simulink model "VisualLocalizationAgent"  (R2024b)
settings: Solver=VariableStepAuto  StartTime=0.0  StopTime=inf  FixedStep=0.05  RelTol=1e-3  EnableMultiTasking=on
undefined symbols (not defined in the file or in its folder): gray, Sim3dSensor
libraries: robotcorelib x2, sim3dcameralib x1, sim3dlib x1, uavsim3dlib x1, uavutilslib x1
settings Model: Creator=The MathWorks, Inc.  LastModifiedBy=vince
settings SolverCC: AlgebraicLoopSolver=TrustRegion  PositivePriorityOrder=on  AutoInsertRateTranBlk=on  MaxZcPerStep=1
settings OptimizationCC: DefaultParameterBehavior=Inlined  EnhancedBackFolding=on  PassReuseOutputArgsAs=Individual arguments  ZeroExternalMemoryAtStartup=off  ZeroInternalMemoryAtStartup=off  MaxStackSize=200000  OptimizeBlockOrder=speed  DifferentSizesBufferReuse=on  OptimizationCustomize=off  EfficientTunableParamExpr=on
settings DebuggingCC: ParameterTunabilityLossMsg=error  UnconnectedInputMsg=warning  UnconnectedOutputMsg=warning  UnconnectedLineMsg=warning  SymbolicDimsDataTypeCodeGenerationDiagnostic=none
settings HardwareCC: ProdBitPerPointer=32  ProdBitPerSizeT=32  ProdBitPerPtrDiffT=32  ProdLargestAtomicInteger=Long  ProdLargestAtomicFloat=Double  ProdWordSize=32  ProdLongLongMode=on  ProdHWDeviceType=ARM Compatible->ARM Cortex-A (32-bit)
settings ModelReferenceCC: EnableRefExpFcnMdlSchedulingChecks=on
settings RTWCC: Description=Embedded Coder  SystemTargetFile=ert.tlc  HardwareBoard=Raspberry Pi  TLCOptions="-aInlineSetEventsForThisBaseRateFcn=TLC_FALSE -aSuppressMultiTaskScheduler=TLC_FALSE  -aRateBasedStepFcn=0"  TemplateMakefile=ert_default_tmf  Toolchain=GNU GCC Embedded Linux  BuildConfiguration=Faster Runs  GPUComputeCapability=3.5  DLArmComputeVersion=19.05
settings CodeAppCC: ForceParamTrailComments=on  IgnoreCustomStorageClasses=off  OperatorAnnotations=on  SimulinkDataObjDesc=on  SFDataObjDesc=on  InsertBlockDesc=on
settings ERTTargetCC: CodeReplacementLibrary=ARM Cortex-A CMSIS  SupportVariableSizeSignals=on  ExtModeTransport=2  ExtModeStaticAlloc=on  ExtModeMexFile=ext_xcp  ExtModeIntrfLevel=Level2 - Open

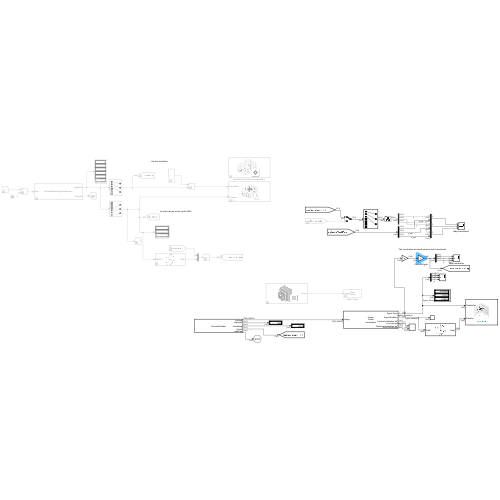
[thumbnail: Simulink's stored preview of the top-level diagram]
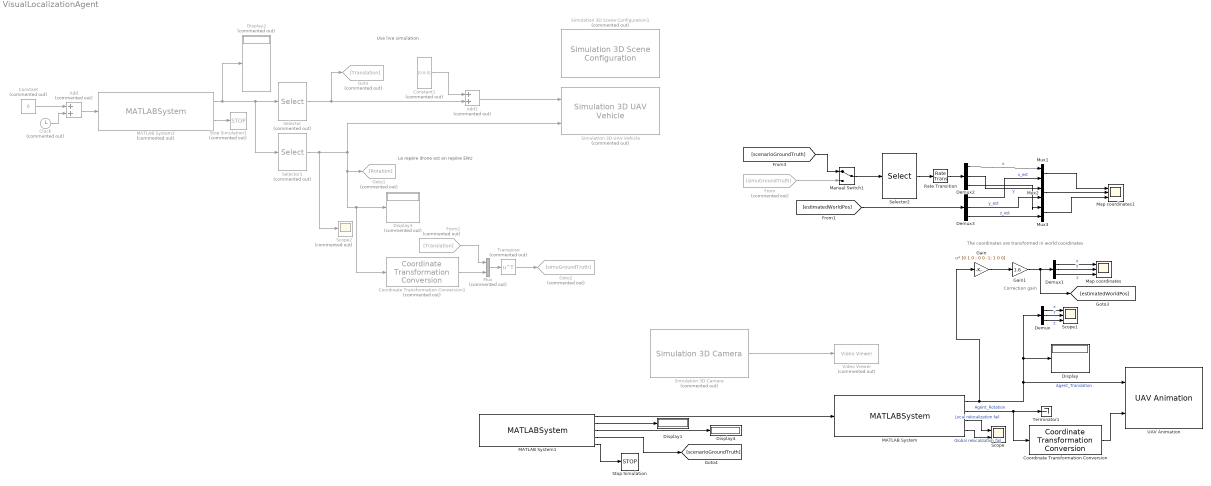
== system VisualLocalizationAgent ==
  note: Correction gain
  note: Use live simulation
  note: The coordinates are transformed in world coordinates
  note: Le repère drone est en repère ENU
  Add : Sum  Commented=on
  Add1 : Sum  Commented=on
  Clock : Clock  Commented=on
  Constant : Constant  Commented=on  Value=0
  Constant1 : Constant  Commented=on  Value=[0;0;0]  VectorParams1D=off
  Coordinate Transformation Conversion : robotcorelib/Coordinate Transformation Conversion  InputRepresentation=Rotation Matrix  InputEulerSequence=ZYX  ShowTrVecInputPort=on  OutputRepresentation=Quaternion  OutputEulerSequence=ZYX  ShowTrVecOutputPort=on  SimulateUsing=Code generation
      settings: LibrarySourceBlock=navlib/Utilities/Coordinate Transformation Conversion
  Coordinate Transformation Conversion1 : robotcorelib/Coordinate Transformation Conversion  Commented=on  InputRepresentation=Euler Angles  InputEulerSequence=ZYX  ShowTrVecInputPort=on  OutputRepresentation=Quaternion  OutputEulerSequence=ZYX  ShowTrVecOutputPort=on  SimulateUsing=Code generation
      settings: LibrarySourceBlock=navlib/Utilities/Coordinate Transformation Conversion
  Demux{,1..3} (4 alike) : Demux  Outputs=3
  Display : Display
  Display1 : Display
  Display2 : Display  Commented=on
  Display3 : Display  Commented=on
  Display4 : Display
  From : From  Commented=on  GotoTag=simuGroundTruth
  From2 : From  Commented=on  GotoTag=Translation
  Gain : Gain  Gain=[0 1 0 ; 0 0 -1; 1 0 0]  Multiplication=Matrix(u*K)
  Gain1 : Gain  Gain=1.6
  Goto : Goto  Commented=on  GotoTag=Translation
  Goto1 : Goto  Commented=on  GotoTag=Rotation
  Goto2 : Goto  Commented=on  GotoTag=simuGroundTruth
  MATLAB System : MATLABSystem  System=Modif_of_HelperVisualLocalizationSystem  FocalLength=[ 1109, 1109 ]  PrincipalPoint=[ 640, 360 ]  ImageSize=[ 720, 1280 ]  ScaleFactor=1.2  NumLevels=8  NumPoints=1500  XLim=[ -15, 40 ]  YLim=[ -10, 5 ]  ZLim=[ -20, 90 ]  SampleTime=-1  ScenariosDirectory=C:\Users\vince\Documents\SEN5\CollaborativeSLAM\Scenarios  ScenarioName=8
      mask Type: Modif_of_HelperVisualLocalizationSystem
      mask Display:
      | disp(['Helper' char(10) 'Visual' char(10) 'Localization']);
      | port_label('input',1,'Image');
      | port_label('output',1,'Agent Pose');
      | port_label('output',2,'Agent Rotation');
      | port_label('output',3,'Local relocalization fail');
      | port_label('output',4,'Global relocalization fail');
  MATLAB System1 : MATLABSystem  System=ScenarioReader  ScenariosDirectory=C:\Users\vince\Documents\SEN5\CollaborativeSLAM\Scenarios  ScenarioName=8  ImageSize=[ 720, 1280, 3 ]  SimulateUsing=Interpreted execution
      mask Type: ScenarioReader
      mask Display:
      | disp('ScenarioReader');
      | port_label('output',1,'currImg');
      | port_label('output',2,'imgIndex');
      | port_label('output',3,'timestamp');
      | port_label('output',4,'gTruth');
      | port_label('output',5,'stopFlag');
  MATLAB System2 : MATLABSystem  Commented=on  System=SmoothBasicWaypointManager  ScenariosDirectory=C:\Users\vince\Documents\SEN5\CollaborativeSLAM\Scenarios  ScenarioName=8  StepTime=0.01  SimulateUsing=Interpreted execution
      mask Type: SmoothBasicWaypointManager
      mask Display:
      | disp('SmoothBasicWaypointManager');
      | port_label('input',1,'time');
      | port_label('output',1,'waypoint');
      | port_label('output',2,'finished');
  Manual Switch1 : ManualSwitch
  Map coordinates : Scope  NumInputPorts=3
  Map coordinates1 : Scope  NumInputPorts=3
  Mux : Mux  Commented=on  Inputs=2
  Mux1 : Mux  Inputs=2
  Mux2 : Mux  Inputs=2
  Mux3 : Mux  Inputs=2
  Rate Transition : RateTransition
  Scope : Scope  NumInputPorts=2
  Scope1 : Scope  NumInputPorts=3
  Scope2 : Scope  Commented=on
  Selector : Selector  Commented=on  InputPortWidth=6  IndexOptions=Index vector (dialog)  Indices=[1 2 3]  OutputSizes=1
  Selector1 : Selector  Commented=on  InputPortWidth=6  IndexOptions=Index vector (dialog)  Indices=[4 5 6]  OutputSizes=1
  Selector2 : Selector  InputPortWidth=7  IndexOptions=Index vector (dialog)  Indices=[1 2 3]  OutputSizes=1
  Simulation 3D Camera : sim3dcameralib/Simulation 3D Camera  Priority=1  Commented=on  sensorTag=Sim3dSensor�  sensorId=1  sensorName=Sim3dSensor�  vehTagList={'Scene Origin';'SimulinkVehicle1'}  vehTag=SimulinkVehicle1  mountLoc=Origin  offsetFlag=on  tmountOffset=[0, 0, 1]  extTmount=off  rmountOffset=[0, 0, 0]  extRmount=off  FocalLength=[1109, 1109]  OpticalCenter=[640, 360]  ImageSize=[720, 1280]  RadialDistortion=[0, 0]  TangentialDistortion=[0, 0]  SensorSkew=0  DepthOutportEnabled=off  SemanticOutportEnabled=off  TransformOutportEnabled=off  SampleTime=1/25  mountPoint=[0 0 1]  mountOrientation=[0 0 0]  aMode=3  ID=1
      settings: LibrarySourceBlock=drivingsim3d/Simulation 3D Camera
  Simulation 3D Scene Configuration1 : sim3dlib/Simulation 3D Scene Configuration  Priority=0  Commented=on  ProjectFormat=Default Scenes  SceneDesc=US city block  ProjectName=C:\Program Files\MATLAB\R2024b\toolbox\shared\sim3d_projects\automotive_project_windows\UE\WindowsNoEditor\VehicleSimulation.exe  ScenePath=/Game/Maps/USCityBlock  EnableOpenDRIVE=off  vehTagList={'Custom';'Scene Origin';'SimulinkVehicle1'}  vehTag=Scene Origin  FreeCameraInitialTranslation=[0, 0, 0]  FreeCameraDefaultInitialTranslation=[-6, 0, 2]  FreeCameraInitialRotation=[0, 0, 0]  FreeCameraDefaultInitialRotation=[0, -15, 0]  OpVisEn=off  Ts=1/100  EnableWindow=on  EnableRemoteAccess=off  EnableWeather=off  SunAzimuth=90  SunAltitude=40.0  EnableGeospatialSun=off  Latitude=0  Longitude=0  Date=2023-01-01  Time=10:30:00  GeoTimeZone=-5.0  SunDaylightSaving=off  wind=1  clouds=10  EnableVolumetricClouds=off  CloudCoverage=0  CloudAltitude=6  fog=0  rain=0  RaindropsEffect=off  SnowDensity=0  EnableGeospatial=off  UseTrueOrigin=off  OriginHeight=200  OriginLatitude=40.744652  OriginLongitude=-73.988864  MapStyle=Aerial  AdditionalAssetIDs=[]  UseAdvancedSunSky=off  SolarTime=11  TimeZone=-5  Day=21  Month=9  Year=2022  UseDaylightSavingTime=on  DSTStartDay=10  DSTStartMonth=3  DSTEndDay=3  DSTEndMonth=11  DSTSwitchHour=2  sensorTag=MainCamera1  sensorId=1  sensorName=Sim3dSensor1  mountLoc=Origin  offsetFlag=off  tmountOffset=[0, 0, 0]  rmountOffset=[0, 0, 0]  HorizontalResolution=1280  VerticalResolution=720  HorizontalFOV=60  mountPoint=[0 0 0]  mountOrientation=[0 0 0]  aMode=4  ID=1  GeoTrigger=Inactive
      settings: LibrarySourceBlock=uavsim3dlib/Simulation 3D Scene Configuration
  Simulation 3D UAV Vehicle : uavsim3dlib/Simulation 3D UAV Vehicle  Priority=-1  Commented=on  Mesh=Quadrotor  MeshPath=/MathWorksUAVContent/UAVs/HexaRotorUAV/HexaRotor.HexaRotor  Color=Black  ActorName=SimulinkVehicle1  UseGlobalFrame=off  InitialTranslation=[0 0 0]  InitialRotation=[0 0 0]  InitialTranslationGlobal=[0 0 0]  InitialGeoOrigin=[0 0 0]  InitialRotationGlobal=[0 0 0]  SampleTime=1/100  ActorType=SimulinkVehicle  ID=1  aMode=4  ActorTag=SimulinkVehicle1
  Stop Simulation : Stop
  Stop Simulation1 : Stop  Commented=on
  Terminator1 : Terminator
  Transpose : Math  Commented=on  Operator=transpose
  UAV Animation : uavutilslib/UAV Animation  NumUAV=1  DynamicUAVConfig=off  UAVType=Multirotor  UAVSize=1  UAVColor=[1 0 0]  UAVTrajectoryAlpha=1  InertialZDirection=Down  RotationFormat=Quaternion  DrawMarkers=off  SampleTime=-1
  Video Viewer : VideoViewer  Commented=on  colormapValue=gray(256)  FigPos=[919 981 958 565]
  wires:
  MATLAB System/2 -> Coordinate Transformation Conversion/1, Terminator1/1  "Agent_Rotation"
  MATLAB System/1 -> UAV Animation/1, Demux/1, Display/1, Gain/1  "Agent_Translation"
  Coordinate Transformation Conversion/1 -> UAV Animation/2
  MATLAB System/3 -> Scope/1  "Local relocalization fail"
  Demux/1 -> Scope1/1  "x"
  Demux/2 -> Scope1/2  "y"
  Demux/3 -> Scope1/3  "z"
  MATLAB System/4 -> Scope/2  "Global relocalization fail"
  MATLAB System1/2 -> Display1/1
  MATLAB System1/5 -> Stop Simulation/1
  Demux1/3 -> Map coordinates/3  "z"
  Demux1/1 -> Map coordinates/1  "x"
  Demux1/2 -> Map coordinates/2  "y"
  Gain/1 -> Gain1/1
  Mux/1 -> Transpose/1
  Add/1 -> MATLAB System2/1
  Clock/1 -> Add/2
  MATLAB System2/2 -> Stop Simulation1/1
  Selector1/1 -> Simulation 3D UAV Vehicle/2, Goto1/1, Coordinate Transformation Conversion1/1, Display3/1, Scope2/1
  Transpose/1 -> Goto2/1
  Selector/1 -> Goto/1, Add1/2
  From2/1 -> Mux/1
  MATLAB System2/1 -> Selector1/1, Selector/1, Display2/1
  Coordinate Transformation Conversion1/1 -> Mux/2
  Constant/1 -> Add/1
  Selector2/1 -> Rate Transition/1
  [estimatedWorldPos] -> Demux3/1
  Demux2/1 -> Mux1/1  "x"
  Demux3/1 -> Mux1/2  "x_est"
  Demux2/2 -> Mux2/1  "y"
  Demux3/2 -> Mux2/2  "y_est"
  Demux3/3 -> Mux3/2  "z_est"
  Demux2/3 -> Mux3/1
  Mux1/1 -> Map coordinates1/1
  Mux2/1 -> Map coordinates1/2
  Mux3/1 -> Map coordinates1/3
  Simulation 3D Camera/1 -> Video Viewer/1
  Rate Transition/1 -> Demux2/1
  [scenarioGroundTruth] -> Manual Switch1/1
  Manual Switch1/1 -> Selector2/1
  MATLAB System1/3 -> Display4/1
  From/1 -> Manual Switch1/2
  Add1/1 -> Simulation 3D UAV Vehicle/1
  Constant1/1 -> Add1/1
  MATLAB System1/1 -> MATLAB System/1
  MATLAB System1/4 -> [scenarioGroundTruth]
  Gain1/1 -> [estimatedWorldPos], Demux1/1
